simulink model "Filter"  (R2020a)
settings: Solver=VariableStepAuto  StartTime=0.0  StopTime=10.0  RelTol=1e-3
settings Model: Creator=HP  LastModifiedBy=HP
settings DataIOCC: SaveOutput=off  SaveTime=off

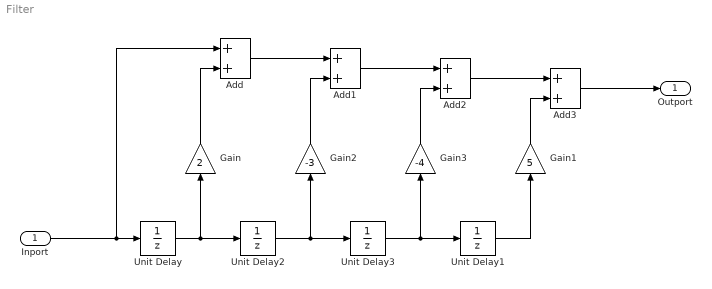
== system Filter ==
  Inport : Inport  OutDataTypeStr=double  PortDimensions=1  SampleTime=[0,1]
  Add{,1..3} (4 alike) : Sum
  Gain : Gain  Gain=2
  Gain1 : Gain  Gain=5
  Gain2 : Gain  Gain=-3
  Gain3 : Gain  Gain=-4
  Unit Delay{,1..3} (4 alike) : UnitDelay  SampleTime=-1  HasFrameUpgradeWarning=on
  Outport : Outport  OutDataTypeStr=double  PortDimensions=1  SampleTime=[0,1]
  wires:
  Unit Delay3/1 -> Gain3/1, Unit Delay1/1
  Inport/1 -> Unit Delay/1, Add/1
  Unit Delay2/1 -> Gain2/1, Unit Delay3/1
  Gain2/1 -> Add1/2
  Add1/1 -> Add2/1
  Unit Delay1/1 -> Gain1/1
  Add2/1 -> Add3/1
  Unit Delay/1 -> Gain/1, Unit Delay2/1
  Gain/1 -> Add/2
  Gain3/1 -> Add2/2
  Gain1/1 -> Add3/2
  Add/1 -> Add1/1
  Add3/1 -> Outport/1
